simulink model "diagrama_de_bloques_actitud"  (R2017b)
settings: Solver=FixedStepDiscrete  StartTime=0.0  StopTime=erle.T_simulacion  FixedStep=erle.Tm  RelTol=1e-3
undefined symbols (not defined in the file or in its folder): erle
settings Model: Creator=javi  LastModifiedBy=javi
settings DataIOCC: SaveFormat=Array

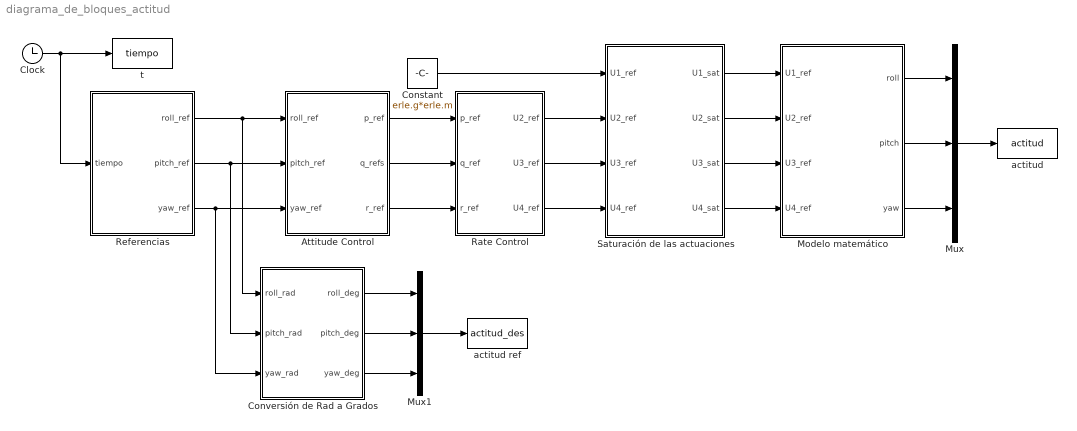
== system diagrama_de_bloques_actitud ==
  Attitude Control : Subsystem
  Clock : Clock
  Constant : Constant  Value=erle.g*erle.m
  Conversión de Rad a Grados : Subsystem
  Modelo matemático : Subsystem
  Mux : Mux  Inputs=3
  Mux1 : Mux  Inputs=3
  Rate Control : Subsystem
  Referencias : Subsystem
  Saturación de las actuaciones : Subsystem
  actitud : ToWorkspace  VariableName=actitud  SampleTime=erle.Tm
  actitud ref : ToWorkspace  VariableName=actitud_des  SampleTime=erle.Tm
  "t " : ToWorkspace  VariableName=tiempo  SampleTime=erle.Tm
  wires:
  Rate Control/1(U2_ref) -> Saturación de las actuaciones/2(U2_ref)
  Rate Control/2(U3_ref) -> Saturación de las actuaciones/3(U3_ref)
  Rate Control/3(U4_ref) -> Saturación de las actuaciones/4(U4_ref)
  Saturación de las actuaciones/1(U1_sat) -> Modelo matemático/1(U1_ref)
  Saturación de las actuaciones/2(U2_sat) -> Modelo matemático/2(U2_ref)
  Saturación de las actuaciones/3(U3_sat) -> Modelo matemático/3(U3_ref)
  Saturación de las actuaciones/4(U4_sat) -> Modelo matemático/4(U4_ref)
  Modelo matemático/1(roll) -> Mux/1
  Modelo matemático/2(pitch) -> Mux/2
  Modelo matemático/3(yaw) -> Mux/3
  Mux/1 -> actitud/1
  Clock/1 -> Referencias/1(tiempo), "t "/1
  Constant/1 -> Saturación de las actuaciones/1(U1_ref)
  Attitude Control/1(p_ref) -> Rate Control/1(p_ref)
  Attitude Control/2(q_refs) -> Rate Control/2(q_ref)
  Attitude Control/3(r_ref) -> Rate Control/3(r_ref)
  Mux1/1 -> actitud ref/1
  Referencias/2(pitch_ref) -> Conversión de Rad a Grados/2(pitch_rad), Attitude Control/2(pitch_ref)
  Conversión de Rad a Grados/3(yaw_deg) -> Mux1/3
  Referencias/3(yaw_ref) -> Attitude Control/3(yaw_ref), Conversión de Rad a Grados/3(yaw_rad)
  Conversión de Rad a Grados/1(roll_deg) -> Mux1/1
  Conversión de Rad a Grados/2(pitch_deg) -> Mux1/2
  Referencias/1(roll_ref) -> Conversión de Rad a Grados/1(roll_rad), Attitude Control/1(roll_ref)

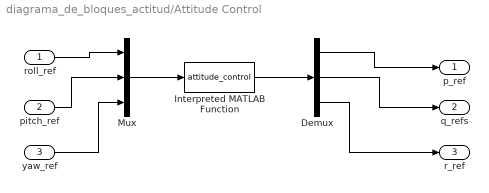
== system diagrama_de_bloques_actitud/Attitude Control ==
  roll_ref : Inport
  pitch_ref : Inport  Port=2
  yaw_ref : Inport  Port=3
  Demux : Demux  Outputs=3
  Interpreted MATLAB Function : MATLABFcn  MATLABFcn=attitude_control  OutputDimensions=3
  Mux : Mux  Inputs=3
  p_ref : Outport
  q_refs : Outport  Port=2
  r_ref : Outport  Port=3
  wires:
  Mux/1 -> Interpreted MATLAB Function/1
  Interpreted MATLAB Function/1 -> Demux/1
  roll_ref/1 -> Mux/1
  pitch_ref/1 -> Mux/2
  yaw_ref/1 -> Mux/3
  Demux/1 -> p_ref/1
  Demux/2 -> q_refs/1
  Demux/3 -> r_ref/1

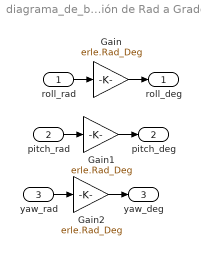
== system diagrama_de_bloques_actitud/Conversión de Rad a Grados ==
  roll_rad : Inport
  pitch_rad : Inport  Port=2
  yaw_rad : Inport  Port=3
  Gain : Gain  Gain=erle.Rad_Deg
  Gain1 : Gain  Gain=erle.Rad_Deg
  Gain2 : Gain  Gain=erle.Rad_Deg
  roll_deg : Outport
  pitch_deg : Outport  Port=2
  yaw_deg : Outport  Port=3
  wires:
  Gain2/1 -> yaw_deg/1
  Gain/1 -> roll_deg/1
  roll_rad/1 -> Gain/1
  yaw_rad/1 -> Gain2/1
  pitch_rad/1 -> Gain1/1
  Gain1/1 -> pitch_deg/1

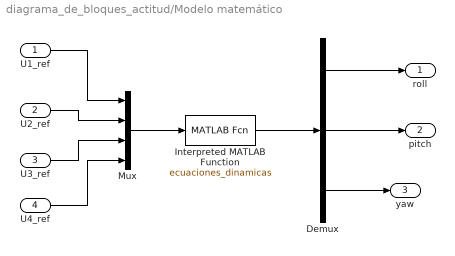
== system diagrama_de_bloques_actitud/Modelo matemático ==
  U1_ref : Inport
  U2_ref : Inport  Port=2
  U3_ref : Inport  Port=3
  U4_ref : Inport  Port=4
  Demux : Demux  Outputs=3
  Interpreted MATLAB Function : MATLABFcn  MATLABFcn=ecuaciones_dinamicas  OutputDimensions=3
  Mux : Mux
  roll : Outport
  pitch : Outport  Port=2
  yaw : Outport  Port=3
  wires:
  U3_ref/1 -> Mux/3
  Mux/1 -> Interpreted MATLAB Function/1
  U2_ref/1 -> Mux/2
  U4_ref/1 -> Mux/4
  U1_ref/1 -> Mux/1
  Interpreted MATLAB Function/1 -> Demux/1
  Demux/1 -> roll/1
  Demux/2 -> pitch/1
  Demux/3 -> yaw/1

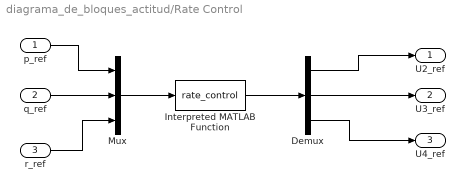
== system diagrama_de_bloques_actitud/Rate Control ==
  p_ref : Inport
  q_ref : Inport  Port=2
  r_ref : Inport  Port=3
  Demux : Demux  Outputs=3
  Interpreted MATLAB Function : MATLABFcn  MATLABFcn=rate_control
  Mux : Mux  Inputs=3
  U2_ref : Outport
  U3_ref : Outport  Port=2
  U4_ref : Outport  Port=3
  wires:
  Demux/3 -> U4_ref/1
  Interpreted MATLAB Function/1 -> Demux/1
  Demux/1 -> U2_ref/1
  q_ref/1 -> Mux/2
  Demux/2 -> U3_ref/1
  p_ref/1 -> Mux/1
  r_ref/1 -> Mux/3
  Mux/1 -> Interpreted MATLAB Function/1

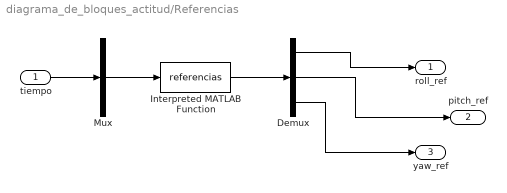
== system diagrama_de_bloques_actitud/Referencias ==
  tiempo : Inport
  Demux : Demux  Outputs=3
  Interpreted MATLAB Function : MATLABFcn  MATLABFcn=referencias
  Mux : Mux  Inputs=1
  roll_ref : Outport
  pitch_ref : Outport  Port=2
  yaw_ref : Outport  Port=3
  wires:
  Mux/1 -> Interpreted MATLAB Function/1
  Interpreted MATLAB Function/1 -> Demux/1
  tiempo/1 -> Mux/1
  Demux/1 -> roll_ref/1
  Demux/2 -> pitch_ref/1
  Demux/3 -> yaw_ref/1

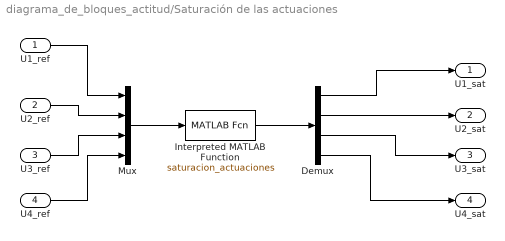
== system diagrama_de_bloques_actitud/Saturación de las actuaciones ==
  U1_ref : Inport
  U2_ref : Inport  Port=2
  U3_ref : Inport  Port=3
  U4_ref : Inport  Port=4
  Demux : Demux
  Interpreted MATLAB Function : MATLABFcn  MATLABFcn=saturacion_actuaciones  OutputDimensions=4
  Mux : Mux
  U1_sat : Outport
  U2_sat : Outport  Port=2
  U3_sat : Outport  Port=3
  U4_sat : Outport  Port=4
  wires:
  Demux/1 -> U1_sat/1
  Interpreted MATLAB Function/1 -> Demux/1
  Demux/2 -> U2_sat/1
  U3_ref/1 -> Mux/3
  Demux/3 -> U3_sat/1
  U4_ref/1 -> Mux/4
  U2_ref/1 -> Mux/2
  U1_ref/1 -> Mux/1
  Demux/4 -> U4_sat/1
  Mux/1 -> Interpreted MATLAB Function/1
